simulink model "Simulink_Car_Model"  (R2021a)
settings: Solver=VariableStepAuto  StartTime=0.0  StopTime=10.0  RelTol=1e-3
model workspace (MAT data in the model file):
  downforce_multiplier = 1
undefined symbols (not defined in the file or in its folder): carData
libraries: sdl_lib x5
settings Model: Creator=eunde  LastModifiedBy=eunde

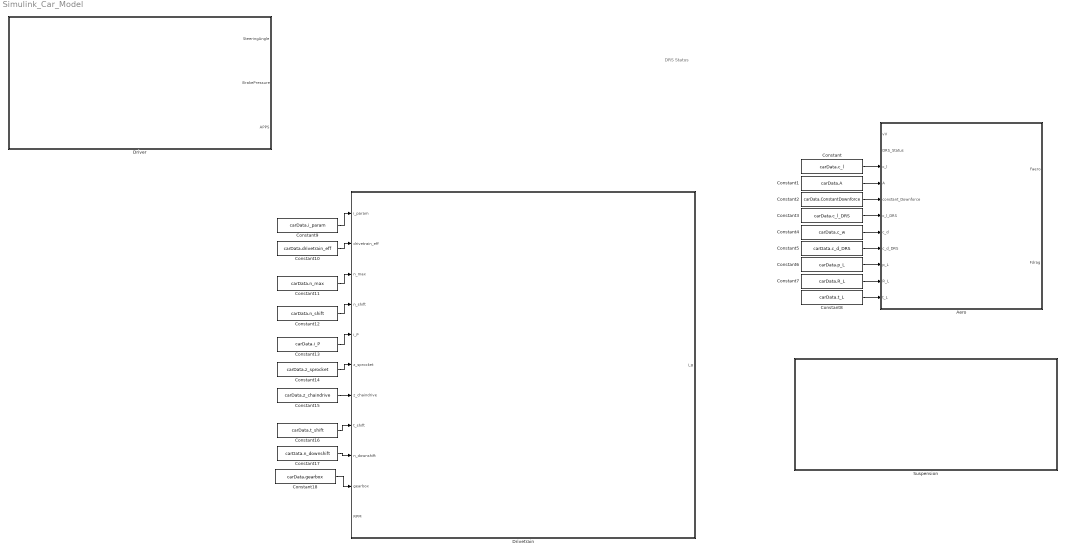
== system Simulink_Car_Model ==
  note: DRS Status
  Aero : Subsystem
  Constant : Constant  Value=carData.c_l
  Constant1 : Constant  Value=carData.A
  Constant10 : Constant  Value=carData.drivetrain_eff
  Constant11 : Constant  Value=carData.n_max
  Constant12 : Constant  Value=carData.n_shift
  Constant13 : Constant  Value=carData.i_P
  Constant14 : Constant  Value=carData.z_sprocket
  Constant15 : Constant  Value=carData.z_chaindrive
  Constant16 : Constant  Value=carData.t_shift
  Constant17 : Constant  Value=carData.n_downshift
  Constant18 : Constant  Value=carData.gearbox
  Constant2 : Constant  Value=carData.ConstantDownforce
  Constant3 : Constant  Value=carData.c_l_DRS
  Constant4 : Constant  Value=carData.c_w
  Constant5 : Constant  Value=carData.c_d_DRS
  Constant6 : Constant  Value=carData.p_L
  Constant7 : Constant  Value=carData.R_L
  Constant8 : Constant  Value=carData.t_L
  Constant9 : Constant  Value=carData.i_param
  Driver : Subsystem
  Drivetrain : Subsystem
  Suspension : Subsystem
  wires:
  Constant/1 -> Aero/3(c_l)
  Constant1/1 -> Aero/4(A)
  Constant2/1 -> Aero/5(constant_Downforce)
  Constant3/1 -> Aero/6(c_l_DRS)
  Constant4/1 -> Aero/7(c_d)
  Constant5/1 -> Aero/8(c_d_DRS)
  Constant6/1 -> Aero/9(p_L)
  Constant7/1 -> Aero/10(R_L)
  Constant8/1 -> Aero/11(t_L)
  Constant9/1 -> Drivetrain/1(i_param)
  Constant10/1 -> Drivetrain/2(drivetrain_eff)
  Constant11/1 -> Drivetrain/3(n_max)
  Constant12/1 -> Drivetrain/4(n_shift)
  Constant13/1 -> Drivetrain/5(i_P)
  Constant14/1 -> Drivetrain/6(z_sprocket)
  Constant15/1 -> Drivetrain/7(z_chaindrive)
  Constant16/1 -> Drivetrain/8(t_shift)
  Constant17/1 -> Drivetrain/9(n_downshift)
  Constant18/1 -> Drivetrain/10(gearbox)

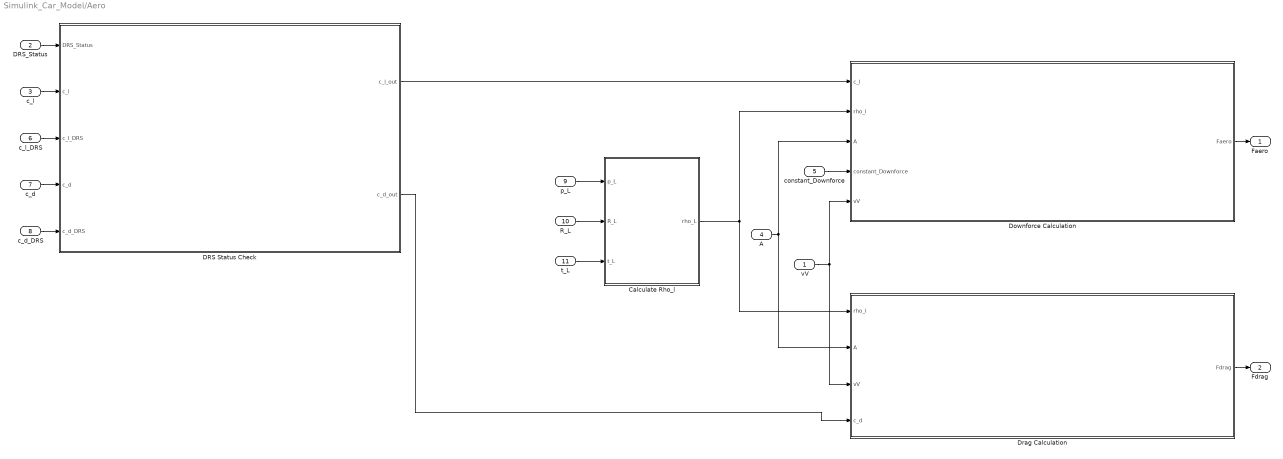
== system Simulink_Car_Model/Aero ==
  vV : Inport
  DRS_Status : Inport  Port=2
  c_l : Inport  Port=3
  A : Inport  Port=4
  constant_Downforce : Inport  Port=5
  c_l_DRS : Inport  Port=6
  c_d : Inport  Port=7
  c_d_DRS : Inport  Port=8
  p_L : Inport  Port=9
  R_L : Inport  Port=10
  t_L : Inport  Port=11
  Calculate Rho_l : Subsystem
  "DRS Status Check " : Subsystem
  Downforce Calculation : Subsystem
  Drag Calculation : Subsystem
  Faero : Outport
  Fdrag : Outport  Port=2
  wires:
  Calculate Rho_l/1(rho_L) -> Downforce Calculation/2(rho_l), Drag Calculation/1(rho_l)
  A/1 -> Downforce Calculation/3(A), Drag Calculation/2(A)
  constant_Downforce/1 -> Downforce Calculation/4(constant_Downforce)
  vV/1 -> Downforce Calculation/5(vV), Drag Calculation/3(vV)
  Downforce Calculation/1(Faero) -> Faero/1
  DRS_Status/1 -> "DRS Status Check "/1(DRS_Status)
  c_l/1 -> "DRS Status Check "/2(c_l)
  c_l_DRS/1 -> "DRS Status Check "/3(c_l_DRS)
  c_d/1 -> "DRS Status Check "/4(c_d)
  c_d_DRS/1 -> "DRS Status Check "/5(c_d_DRS)
  "DRS Status Check "/1(c_l_out) -> Downforce Calculation/1(c_l)
  "DRS Status Check "/2(c_d_out) -> Drag Calculation/4(c_d)
  Drag Calculation/1(Fdrag) -> Fdrag/1
  p_L/1 -> Calculate Rho_l/1(p_L)
  R_L/1 -> Calculate Rho_l/2(R_L)
  t_L/1 -> Calculate Rho_l/3(t_L)

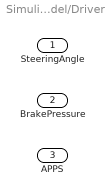
== system Simulink_Car_Model/Driver ==
  SteeringAngle : Outport
  BrakePressure : Outport  Port=2
  APPS : Outport  Port=3

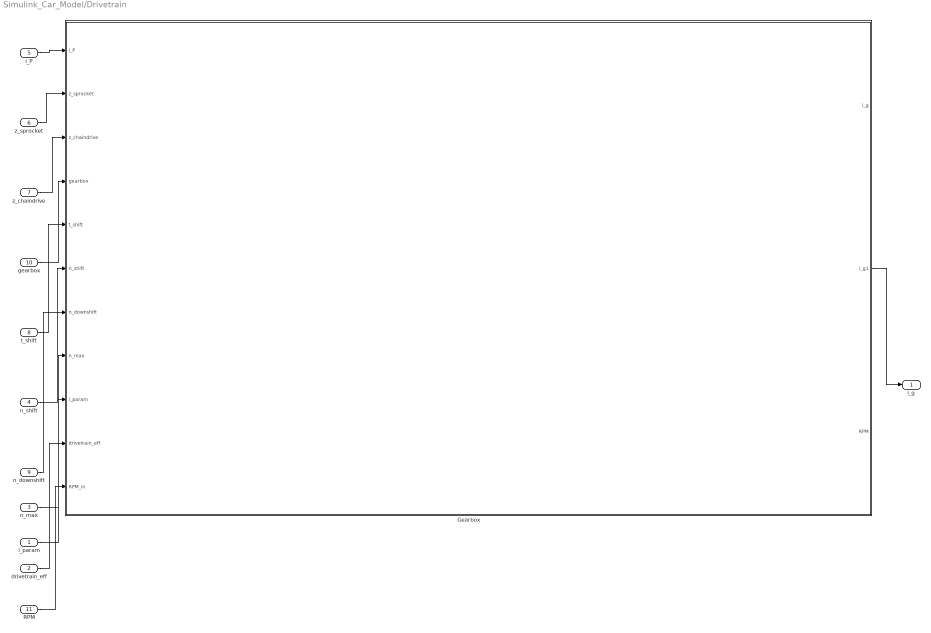
== system Simulink_Car_Model/Drivetrain ==
  i_param : Inport
  drivetrain_eff : Inport  Port=2
  n_max : Inport  Port=3
  n_shift : Inport  Port=4
  i_P : Inport  Port=5
  z_sprocket : Inport  Port=6
  z_chaindrive : Inport  Port=7
  t_shift : Inport  Port=8
  n_downshift : Inport  Port=9
  gearbox : Inport  Port=10
  RPM : Inport  Port=11
  Gearbox : Subsystem
  i_g : Outport
  wires:
  i_P/1 -> Gearbox/1(i_P)
  z_sprocket/1 -> Gearbox/2(z_sprocket)
  z_chaindrive/1 -> Gearbox/3(z_chaindrive)
  gearbox/1 -> Gearbox/4(gearbox)
  Gearbox/2(i_g1) -> i_g/1
  t_shift/1 -> Gearbox/5(t_shift)
  n_shift/1 -> Gearbox/6(n_shift)
  n_downshift/1 -> Gearbox/7(n_downshift)
  n_max/1 -> Gearbox/8(n_max)
  i_param/1 -> Gearbox/9(i_param)
  drivetrain_eff/1 -> Gearbox/10(drivetrain_eff)
  RPM/1 -> Gearbox/11(RPM_in)

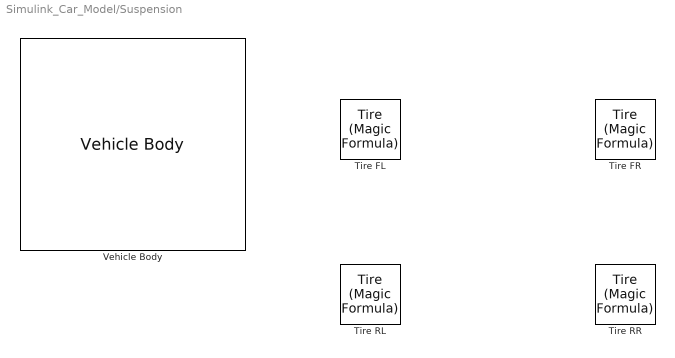
== system Simulink_Car_Model/Suspension ==
  Tire FL : sdl_lib/Tires & Vehicles/Tire (Magic Formula)  parameterization=sdl.enum.magic_tire_model.load  F_z1=3000 N  F_x1=3500 N  kappa1=10  B_m=10  C_m=1.9  D_m=1  E_m=0.97  fz0=4000 N  p_Cx=1.685  p_Dx=[1.21, -.037]  p_Ex=[.344, .095, -.02, 0]  p_Kx=[21.51, -.163, .245]  p_Hx=[-.002, .002]  p_Vx=[0, 0]  v_tr_thr=0.1 m/s  r_e=0.3 m  model_compliance=1  stiffness=1e6 N/m  damping=1000 N/(m/s)  model_inertia=1  inertia=1 kg*m^2  initial_velocity=0 rad/s  model_resistance=1  resistance_model=1  coeff=0.015  p_tire=250e3 Pa  alpha=-0.003  beta=0.97  coeff_a=84e-4  coeff_b=6.2e-4 s/m  coeff_c=1.6e-4 s^2/m^2  v_thr=0.001 m/s
  Tire FR : sdl_lib/Tires & Vehicles/Tire (Magic Formula)  parameterization=sdl.enum.magic_tire_model.load  F_z1=3000 N  F_x1=3500 N  kappa1=10  B_m=10  C_m=1.9  D_m=1  E_m=0.97  fz0=4000 N  p_Cx=1.685  p_Dx=[1.21, -.037]  p_Ex=[.344, .095, -.02, 0]  p_Kx=[21.51, -.163, .245]  p_Hx=[-.002, .002]  p_Vx=[0, 0]  v_tr_thr=0.1 m/s  r_e=0.3 m  model_compliance=1  stiffness=1e6 N/m  damping=1000 N/(m/s)  model_inertia=1  inertia=1 kg*m^2  initial_velocity=0 rad/s  model_resistance=1  resistance_model=1  coeff=0.015  p_tire=250e3 Pa  alpha=-0.003  beta=0.97  coeff_a=84e-4  coeff_b=6.2e-4 s/m  coeff_c=1.6e-4 s^2/m^2  v_thr=0.001 m/s
  Tire RL : sdl_lib/Tires & Vehicles/Tire (Magic Formula)  parameterization=sdl.enum.magic_tire_model.load  F_z1=3000 N  F_x1=3500 N  kappa1=10  B_m=10  C_m=1.9  D_m=1  E_m=0.97  fz0=4000 N  p_Cx=1.685  p_Dx=[1.21, -.037]  p_Ex=[.344, .095, -.02, 0]  p_Kx=[21.51, -.163, .245]  p_Hx=[-.002, .002]  p_Vx=[0, 0]  v_tr_thr=0.1 m/s  r_e=0.3 m  model_compliance=1  stiffness=1e6 N/m  damping=1000 N/(m/s)  model_inertia=1  inertia=1 kg*m^2  initial_velocity=0 rad/s  model_resistance=1  resistance_model=1  coeff=0.015  p_tire=250e3 Pa  alpha=-0.003  beta=0.97  coeff_a=84e-4  coeff_b=6.2e-4 s/m  coeff_c=1.6e-4 s^2/m^2  v_thr=0.001 m/s
  Tire RR : sdl_lib/Tires & Vehicles/Tire (Magic Formula)  parameterization=sdl.enum.magic_tire_model.load  F_z1=3000 N  F_x1=3500 N  kappa1=10  B_m=10  C_m=1.9  D_m=1  E_m=0.97  fz0=4000 N  p_Cx=1.685  p_Dx=[1.21, -.037]  p_Ex=[.344, .095, -.02, 0]  p_Kx=[21.51, -.163, .245]  p_Hx=[-.002, .002]  p_Vx=[0, 0]  v_tr_thr=0.1 m/s  r_e=0.3 m  model_compliance=1  stiffness=1e6 N/m  damping=1000 N/(m/s)  model_inertia=1  inertia=1 kg*m^2  initial_velocity=0 rad/s  model_resistance=1  resistance_model=1  coeff=0.015  p_tire=250e3 Pa  alpha=-0.003  beta=0.97  coeff_a=84e-4  coeff_b=6.2e-4 s/m  coeff_c=1.6e-4 s^2/m^2  v_thr=0.001 m/s
  Vehicle Body : sdl_lib/Tires & Vehicles/Vehicle Body  mass=200 kg  n_w=2  x_f=1.4 m  x_r=1.6 m  y_c=0.5 m  mass_var=simscape.enum.onoff.off  model_pitch=simscape.enum.onoff.off  inertia=4000 kg*m^2  suspension_model=sdl.enum.linearTLU.linear  k_f=1e4 N/m  b_f=1e4 N/(m/s)  k_r=1e4 N/m  b_r=1e4 N/(m/s)  k_f_TLU=[-2000, -1000, 0, 1000, 2000] N  x_f_TLU=[-.4, -.2, 0, .2, .4] m  b_f_TLU=[-200, -100, 0, 100, 200] N  v_f_TLU=[-4, -2, 0, 2, 4] m/s  k_r_TLU=[-2000, -1000, 0, 1000, 2000] N  x_r_TLU=[-.4, -.2, 0, .2, .4] m  b_r_TLU=[-200, -100, 0, 100, 200] N  v_r_TLU=[-4, -2, 0, 2, 4] m/s  interp_method=simscape.enum.interpolation.linear  extrap_method=simscape.enum.extrapolation.linear  model_hardstop=simscape.enum.onoff.off  upper_bound_f=.25 m  lower_bound_f=-.25 m  stop_k_f=1e6 N/m  stop_b_f=150 N/(m/s)  upper_bound_r=.25 m  lower_bound_r=-.25 m  stop_k_r=1e6 N/m  stop_b_r=150 N/(m/s)  initial_pitch=0 rad  initial_pitch_rate=0 rad/s  g=9.81 m/s^2  liftoff_warning=simscape.enum.onoff.off  area=3 m^2  Cd=0.4  rho=1.18 kg/m^3  v_specify=off  v_priority=High  v=0 m/s  v_nominal_specify=off  v_nominal_unit=m/s  v_nominal_value=1

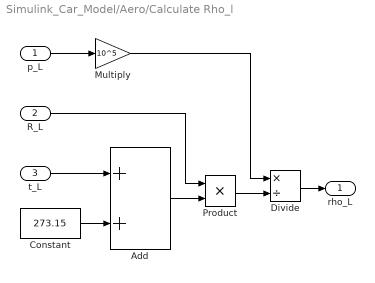
== system Simulink_Car_Model/Aero/Calculate Rho_l ==
  p_L : Inport
  R_L : Inport  Port=2
  t_L : Inport  Port=3
  Add : Sum
  Constant : Constant  Value=273.15
  Divide : Product  Inputs=*/
  Multiply : Gain  Gain=10^5
  Product : Product
  rho_L : Outport
  wires:
  p_L/1 -> Multiply/1
  t_L/1 -> Add/1
  Constant/1 -> Add/2
  Add/1 -> Product/2
  R_L/1 -> Product/1
  Multiply/1 -> Divide/1
  Product/1 -> Divide/2
  Divide/1 -> rho_L/1

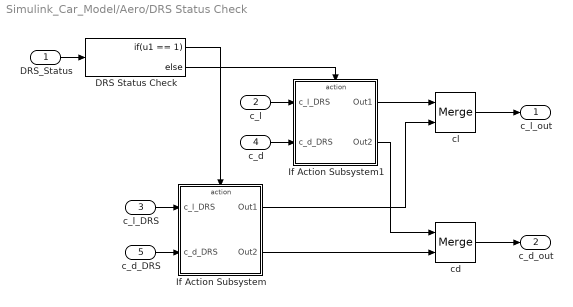
== system Simulink_Car_Model/Aero/DRS Status Check  ==
  DRS_Status : Inport
  c_l : Inport  Port=2
  c_l_DRS : Inport  Port=3
  c_d : Inport  Port=4
  c_d_DRS : Inport  Port=5
  DRS Status Check : If  IfExpression=u1 == 1
  If Action Subsystem : Subsystem  TreatAsAtomicUnit=on
  If Action Subsystem1 : Subsystem  TreatAsAtomicUnit=on
  cd : Merge
  cl : Merge
  c_l_out : Outport
  c_d_out : Outport  Port=2
  wires:
  c_l_DRS/1 -> If Action Subsystem/1(c_l_DRS)
  If Action Subsystem1/2(Out2) -> cd/1
  c_l/1 -> If Action Subsystem1/1(c_l_DRS)
  If Action Subsystem1/1(Out1) -> cl/1
  c_d_DRS/1 -> If Action Subsystem/2(c_d_DRS)
  DRS Status Check/2 -> If Action Subsystem1/Action
  cl/1 -> c_l_out/1
  If Action Subsystem/1(Out1) -> cl/2
  DRS_Status/1 -> DRS Status Check/1
  DRS Status Check/1 -> If Action Subsystem/Action
  If Action Subsystem/2(Out2) -> cd/2
  c_d/1 -> If Action Subsystem1/2(c_d_DRS)
  cd/1 -> c_d_out/1

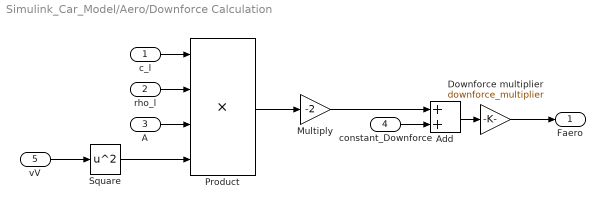
== system Simulink_Car_Model/Aero/Downforce Calculation ==
  c_l : Inport
  rho_l : Inport  Port=2
  A : Inport  Port=3
  constant_Downforce : Inport  Port=4
  vV : Inport  Port=5
  Add : Sum
  Downforce multiplier : Gain  Gain=downforce_multiplier
  Multiply : Gain  Gain=-2
  Product : Product  Inputs=4
  Square : Math  Operator=square  SaturateOnIntegerOverflow=on
  Faero : Outport
  wires:
  vV/1 -> Square/1
  A/1 -> Product/3
  rho_l/1 -> Product/2
  Downforce multiplier/1 -> Faero/1
  Add/1 -> Downforce multiplier/1
  constant_Downforce/1 -> Add/2
  Product/1 -> Multiply/1
  Multiply/1 -> Add/1
  Square/1 -> Product/4
  c_l/1 -> Product/1

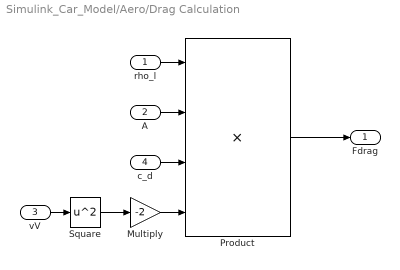
== system Simulink_Car_Model/Aero/Drag Calculation ==
  rho_l : Inport
  A : Inport  Port=2
  vV : Inport  Port=3
  c_d : Inport  Port=4
  Multiply : Gain  Gain=-2
  Product : Product  Inputs=4
  Square : Math  Operator=square  SaturateOnIntegerOverflow=on
  Fdrag : Outport
  wires:
  vV/1 -> Square/1
  Square/1 -> Multiply/1
  rho_l/1 -> Product/1
  A/1 -> Product/2
  c_d/1 -> Product/3
  Multiply/1 -> Product/4
  Product/1 -> Fdrag/1

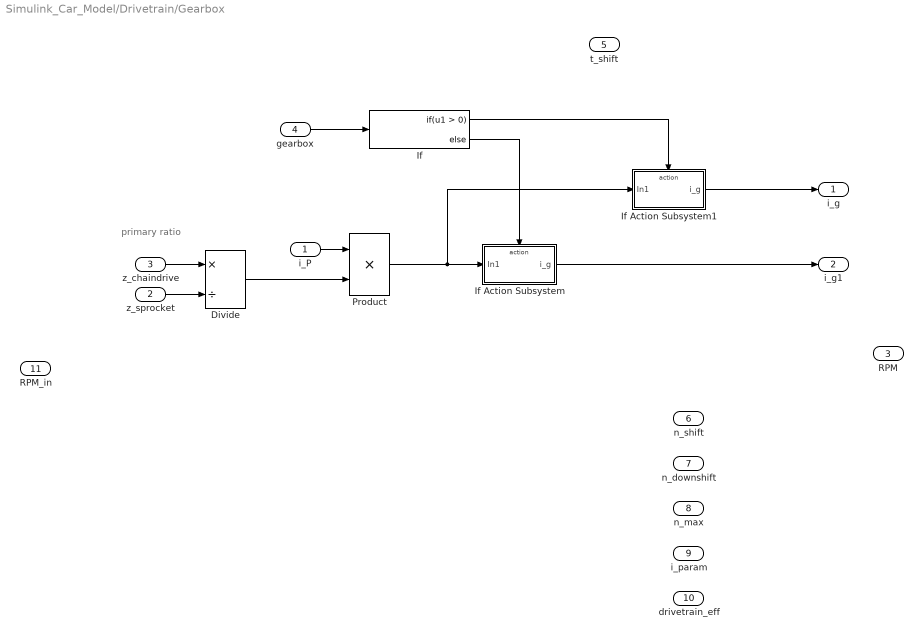
== system Simulink_Car_Model/Drivetrain/Gearbox ==
  note: primary ratio
  i_P : Inport
  z_sprocket : Inport  Port=2
  z_chaindrive : Inport  Port=3
  gearbox : Inport  Port=4
  t_shift : Inport  Port=5
  n_shift : Inport  Port=6
  n_downshift : Inport  Port=7
  n_max : Inport  Port=8
  i_param : Inport  Port=9
  drivetrain_eff : Inport  Port=10
  RPM_in : Inport  Port=11
  Divide : Product  Inputs=*/
  If : If
  If Action Subsystem : Subsystem  TreatAsAtomicUnit=on
  If Action Subsystem1 : Subsystem  TreatAsAtomicUnit=on
  Product : Product
  i_g : Outport
  i_g1 : Outport  Port=2
  RPM : Outport  Port=3
  wires:
  If/1 -> If Action Subsystem1/Action
  i_P/1 -> Product/1
  If/2 -> If Action Subsystem/Action
  z_sprocket/1 -> Divide/2
  Divide/1 -> Product/2
  If Action Subsystem/1(i_g) -> i_g1/1
  Product/1 -> If Action Subsystem1/1(In1), If Action Subsystem/1(In1)
  z_chaindrive/1 -> Divide/1
  gearbox/1 -> If/1
  If Action Subsystem1/1(i_g) -> i_g/1

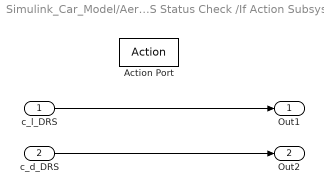
== system Simulink_Car_Model/Aero/DRS Status Check /If Action Subsystem ==
  c_l_DRS : Inport
  c_d_DRS : Inport  Port=2
  Action Port : ActionPort  ActionPortLabel=if(u1 == 1)
  Out1 : Outport
  Out2 : Outport  Port=2
  wires:
  c_l_DRS/1 -> Out1/1
  c_d_DRS/1 -> Out2/1

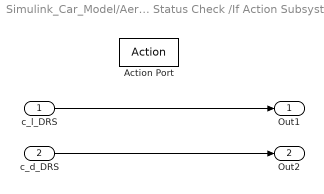
== system Simulink_Car_Model/Aero/DRS Status Check /If Action Subsystem1 ==
  c_l_DRS : Inport
  c_d_DRS : Inport  Port=2
  Action Port : ActionPort  ActionPortLabel=else
  Out1 : Outport
  Out2 : Outport  Port=2
  wires:
  c_l_DRS/1 -> Out1/1
  c_d_DRS/1 -> Out2/1

== system Simulink_Car_Model/Drivetrain/Gearbox/If Action Subsystem ==
  In1 : Inport
  Action Port : ActionPort  ActionPortLabel=else
  i_g : Outport
  wires:
  In1/1 -> i_g/1

== system Simulink_Car_Model/Drivetrain/Gearbox/If Action Subsystem1 ==
  In1 : Inport
  Action Port : ActionPort  ActionPortLabel=if(u1 > 0)
  i_g : Outport
  wires:
  In1/1 -> i_g/1
